simulink model "IMSPM_Q36121333_LAB4_SYSTEM_hybrid"  (R2021b)
settings: Solver=ode45  StartTime=0.0  StopTime=0.015  MaxStep=1e-8  RelTol=1e-3
undefined symbols (not defined in the file): plecs
libraries: simulink x1, modelsimlib x1
settings Model: Creator=stanl  LastModifiedBy=stanl

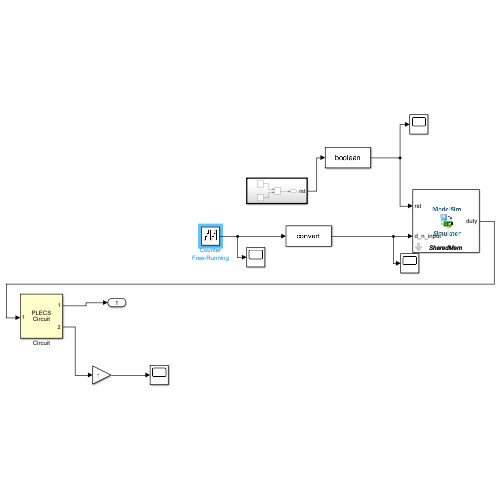
[thumbnail: Simulink's stored preview of the top-level diagram]
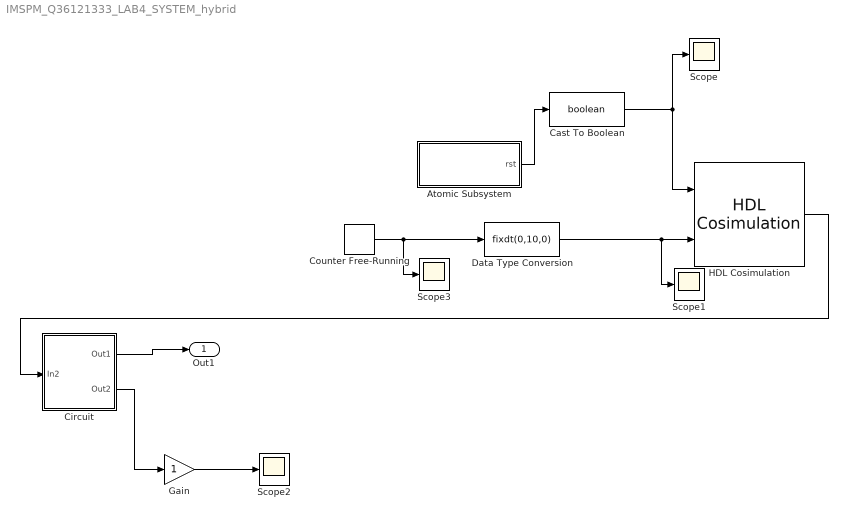
== system IMSPM_Q36121333_LAB4_SYSTEM_hybrid ==
  Atomic Subsystem : Subsystem  TreatAsAtomicUnit=on
  Cast To Boolean : DataTypeConversion  OutDataTypeStr=boolean
  Circuit : Subsystem  LoadFcn=plecs('sl', 200);  InitFcn=plecs('sl', 214);  StartFcn=plecs('sl', 208);  StopFcn=plecs('sl', 209);  mask(PlecsCircuit){PLECSData=<binary blob, 3008 chars, not shown>}
      mask prompts: PLECSData "PLECS Data (Do not delete or modify!)"
      mask init:
      | % PLACE CUSTOM INITIALIZATIONS ABOVE
      | % DO NOT REMOVE
      | plecs('sl', 215);
      | % DO NOT REMOVE
      settings: CopyFcn=plecs('sl', 203);  DeleteFcn=plecs('sl', 205);  UndoDeleteFcn=plecs('sl', 206);  PreSaveFcn=plecs('sl', 211);  PostSaveFcn=plecs('sl', 201);  NameChangeFcn=plecs('sl', 210);  DestroyFcn=plecs('sl', 207);  PreCopyFcn=plecs('sl', 216);  OpenFcn=plecs('sl', 202);  ErrorFcn=plerrorfcn
      mask Help: web(['file:///' fullfile(plecsdoc, 'creatingacircuit.html')])
      mask Display: disp('PLECS\nCircuit')
  Counter Free-Running : simulink/Sources/Counter Free-Running  NumBits=10  tsamp=1e-3
  Data Type Conversion : DataTypeConversion  OutDataTypeStr=fixdt(0,10,0)
  Gain : Gain
  HDL Cosimulation : modelsimlib/HDL Cosimulation  PortPaths=/hybrid_pwm/rst;/hybrid_pwm/d_n_input;/hybrid_pwm/duty  PortModes=[1 1 2 ]  PortTimes=[-1,-1,5e-9]  PortSigns=[-1 -1 -1 ]  PortFracLengths=[0,0,0]  CommLocal=on  CommSharedMemory=on  CommPortNumber=4449  CommShowInfo=on  ClockPaths=/hybrid_pwm/clk_count  ClockModes=[2 ]  ClockTimes=[2e-8]  TclPreSimCommand="puts \"Running Simulink Cosimulation block.\""  TclPostSimCommand="puts \"done\""  TimingMode=s  TimingScaleFactor=1  idxCellArray={'UNUSED_VAR'}  CosimBypass=Full Simulation  AllowDirectFeedthrough=on  ProductName=EDA Simulator Link MQ  RunAutoTimescale=off  HdlClocks=0  PreRunTime=0  PreRunTimeUnit=ns
      settings: SourceProductBaseCode=ES
  Scope{,1..3} (4 alike) : Scope
  Out1 : Outport
  wires:
  Counter Free-Running/1 -> Scope3/1, Data Type Conversion/1
  Cast To Boolean/1 -> HDL Cosimulation/1, Scope/1
  Atomic Subsystem/1(rst) -> Cast To Boolean/1
  Circuit/1(Out1) -> Out1/1
  Gain/1 -> Scope2/1
  Data Type Conversion/1 -> HDL Cosimulation/2, Scope1/1
  Circuit/2(Out2) -> Gain/1
  HDL Cosimulation/1 -> Circuit/1(In2)

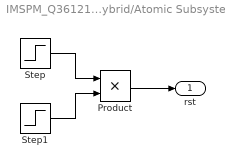
== system IMSPM_Q36121333_LAB4_SYSTEM_hybrid/Atomic Subsystem ==
  Product : Product
  Step : Step  Time=0.5e-6  SampleTime=1e-8
  Step1 : Step  Time=0.8e-6  Before=1  After=0  SampleTime=1e-8
  rst : Outport
  wires:
  Step1/1 -> Product/2
  Step/1 -> Product/1
  Product/1 -> rst/1

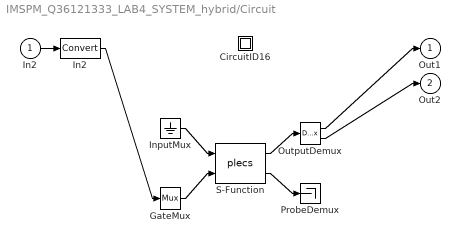
== system IMSPM_Q36121333_LAB4_SYSTEM_hybrid/Circuit ==
  In2 : Inport  PortDimensions=1
  " CircuitID16 " : Subsystem
  " GateMux " : Mux  Inputs=[ 1 ]
  " In2 " : DataTypeConversion  SaturateOnIntegerOverflow=on  RndMeth=Zero
  " InputMux " : Ground
  " OutputDemux " : Demux  Outputs=[ 1 1 ]
  " ProbeDemux " : Terminator
  " S-Function " : S-Function  FunctionName=plecs  SFunctionDeploymentMode=off  EnableBusSupport=off
  Out1 : Outport  PortDimensions=1
  Out2 : Outport  Port=2  PortDimensions=1
  wires:
  " InputMux "/1 -> " S-Function "/1
  " GateMux "/1 -> " S-Function "/2
  " S-Function "/1 -> " OutputDemux "/1
  " S-Function "/2 -> " ProbeDemux "/1
  In2/1 -> " In2 "/1
  " In2 "/1 -> " GateMux "/1
  " OutputDemux "/1 -> Out1/1
  " OutputDemux "/2 -> Out2/1

== system IMSPM_Q36121333_LAB4_SYSTEM_hybrid/Circuit/ CircuitID16  ==
